simulink model "process_test_windup_2015"  (R2015a)
settings: Solver=ode45  SolverMode=SingleTasking  StartTime=0.0  StopTime=5000  RelTol=1e-3
libraries: simulink x4
settings Model: CovMetricSettings=dwe  CovHtmlReporting=off  covSaveCumulativeToWorkspaceVar=off  CovSaveSingleToWorkspaceVar=off  CovExternalEMLEnable=on  Creator=Bailey Brookes  LastModifiedBy=Bailey Brookes
settings DataIOCC: LimitDataPoints=off  SaveFormat=Dataset
settings OptimizationCC: InlineParams=on  BufferReuse=off
settings DebuggingCC: InitInArrayFormatMsg=none  SFUnexpectedBacktrackingDiag=error  SFNoUnconditionalDefaultTransitionDiag=error
settings HardwareCC: ProdBitPerPointer=64  ProdLargestAtomicFloat=Float  ProdIntDivRoundTo=Zero  ProdEndianess=LittleEndian  ProdHWDeviceType=Specified
settings ModelReferenceCC: PropagateSignalLabelsOutOfModel=on
settings GRTTargetCC: TargetLangStandard=C99 (ISO)  GeneratePreprocessorConditionals=Use local settings

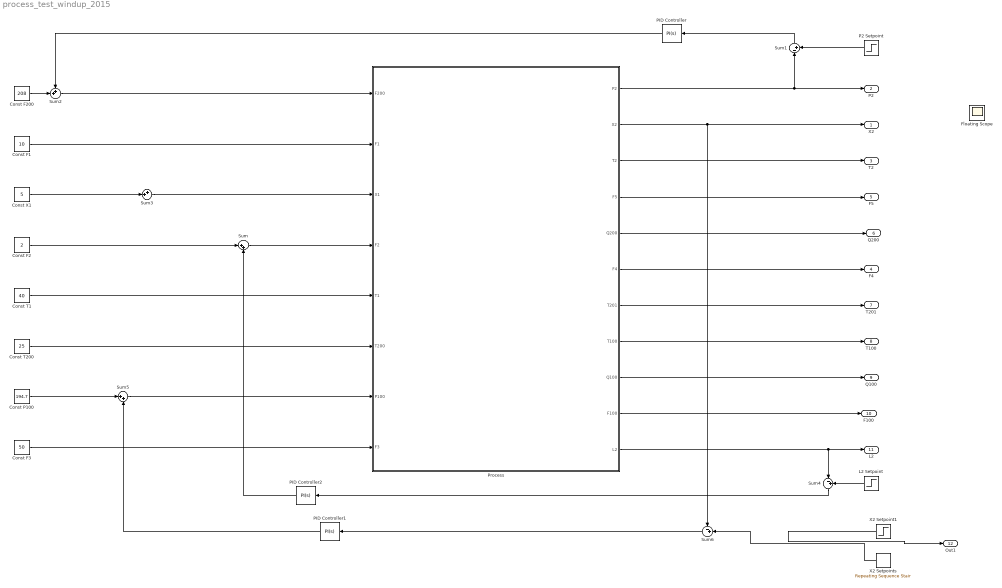
== system process_test_windup_2015 ==
  Const F1 : Constant  Value=10
  Const F2 : Constant  Value=2
  Const F200 : Constant  Value=208
  Const F3 : Constant  Value=50
  Const P100 : Constant  Value=194.7
  Const T1 : Constant  Value=40
  Const T200 : Constant  Value=25
  Const X1 : Constant  Value=5
  Floating Scope : Scope
      settings: Floating=on  TimeRange=auto  MaxDataPoints=5000  SaveToWorkspace=off  SaveName=ScopeData  YMin=-10.40191  YMax=93.61723  SampleTime=-1
  L2 Setpoint : Step  Before=1  After=1.4  SampleTime=0
  P2 Setpoint : Step  Before=50.5  After=50.5  SampleTime=0
  PID Controller : simulink/Continuous/PID Controller  Controller=PI  TimeDomain=Continuous-time  SampleTime=-1  IntegratorMethod=Forward Euler  FilterMethod=Forward Euler  Form=Parallel  UseFilter=on  ControllerParametersSource=internal  P=-803.5  I=-803.5/12  D=0  N=100  InitialConditionSource=internal  InitialConditionForIntegrator=0  InitialConditionForFilter=0  ExternalReset=none  LimitOutput=on  UpperSaturationLimit=208  LowerSaturationLimit=-208  LinearizeAsGain=on  AntiWindupMode=clamping  Kb=1  TrackingMode=off  Kt=1  PParamMin=[]  PParamMax=[]  IParamMin=[]  IParamMax=[]  DParamMin=[]  DParamMax=[]  NParamMin=[]  NParamMax=[]  KbParamMin=[]  KbParamMax=[]  KtParamMin=[]  KtParamMax=[]  POutMin=[]  POutMax=[]  IOutMin=[]  IOutMax=[]  DOutMin=[]  DOutMax=[]  NOutMin=[]  NOutMax=[]  KbOutMin=[]  KbOutMax=[]  KtOutMin=[]  KtOutMax=[]  IntegratorOutMin=[]  IntegratorOutMax=[]  FilterOutMin=[]  FilterOutMax=[]  SumOutMin=[]  SumOutMax=[]  SumI1OutMin=[]  SumI1OutMax=[]  SumI2OutMin=[]  SumI2OutMax=[]  SumI3OutMin=[]  SumI3OutMax=[]  SumDOutMin=[]  SumDOutMax=[]  SaturationOutMin=[]  SaturationOutMax=[]  IntegratorContinuousStateAttributes=''  IntegratorStateMustResolveToSignalObject=off  IntegratorRTWStateStorageClass=Auto  FilterContinuousStateAttributes=''  FilterStateMustResolveToSignalObject=off  FilterRTWStateStorageClass=Auto  DifferentiatorICPrevScaledInput=0  DifferentiatorOutMin=[]  DifferentiatorOutMax=[]
  PID Controller1 : simulink/Continuous/PID Controller  Controller=PI  TimeDomain=Continuous-time  SampleTime=-1  IntegratorMethod=Forward Euler  FilterMethod=Forward Euler  Form=Parallel  UseFilter=on  ControllerParametersSource=internal  P=4.41  I=4.41*1.2/17.7  D=0  N=100  InitialConditionSource=internal  InitialConditionForIntegrator=0  InitialConditionForFilter=0  ExternalReset=none  LimitOutput=on  UpperSaturationLimit=194.7  LowerSaturationLimit=-194.7  LinearizeAsGain=on  AntiWindupMode=clamping  Kb=1  TrackingMode=off  Kt=1  PParamMin=[]  PParamMax=[]  IParamMin=[]  IParamMax=[]  DParamMin=[]  DParamMax=[]  NParamMin=[]  NParamMax=[]  KbParamMin=[]  KbParamMax=[]  KtParamMin=[]  KtParamMax=[]  POutMin=[]  POutMax=[]  IOutMin=[]  IOutMax=[]  DOutMin=[]  DOutMax=[]  NOutMin=[]  NOutMax=[]  KbOutMin=[]  KbOutMax=[]  KtOutMin=[]  KtOutMax=[]  IntegratorOutMin=[]  IntegratorOutMax=[]  FilterOutMin=[]  FilterOutMax=[]  SumOutMin=[]  SumOutMax=[]  SumI1OutMin=[]  SumI1OutMax=[]  SumI2OutMin=[]  SumI2OutMax=[]  SumI3OutMin=[]  SumI3OutMax=[]  SumDOutMin=[]  SumDOutMax=[]  SaturationOutMin=[]  SaturationOutMax=[]  IntegratorContinuousStateAttributes=''  IntegratorStateMustResolveToSignalObject=off  IntegratorRTWStateStorageClass=Auto  FilterContinuousStateAttributes=''  FilterStateMustResolveToSignalObject=off  FilterRTWStateStorageClass=Auto  DifferentiatorICPrevScaledInput=0  DifferentiatorOutMin=[]  DifferentiatorOutMax=[]
  PID Controller2 : simulink/Continuous/PID Controller  Controller=PI  TimeDomain=Continuous-time  SampleTime=-1  IntegratorMethod=Forward Euler  FilterMethod=Forward Euler  Form=Parallel  UseFilter=on  ControllerParametersSource=internal  P=-13.9  I=-13.9/19.2  D=0  N=100  InitialConditionSource=internal  InitialConditionForIntegrator=0  InitialConditionForFilter=0  ExternalReset=none  LimitOutput=on  UpperSaturationLimit=2  LowerSaturationLimit=-2  LinearizeAsGain=on  AntiWindupMode=clamping  Kb=1  TrackingMode=off  Kt=1  PParamMin=[]  PParamMax=[]  IParamMin=[]  IParamMax=[]  DParamMin=[]  DParamMax=[]  NParamMin=[]  NParamMax=[]  KbParamMin=[]  KbParamMax=[]  KtParamMin=[]  KtParamMax=[]  POutMin=[]  POutMax=[]  IOutMin=[]  IOutMax=[]  DOutMin=[]  DOutMax=[]  NOutMin=[]  NOutMax=[]  KbOutMin=[]  KbOutMax=[]  KtOutMin=[]  KtOutMax=[]  IntegratorOutMin=[]  IntegratorOutMax=[]  FilterOutMin=[]  FilterOutMax=[]  SumOutMin=[]  SumOutMax=[]  SumI1OutMin=[]  SumI1OutMax=[]  SumI2OutMin=[]  SumI2OutMax=[]  SumI3OutMin=[]  SumI3OutMax=[]  SumDOutMin=[]  SumDOutMax=[]  SaturationOutMin=[]  SaturationOutMax=[]  IntegratorContinuousStateAttributes=''  IntegratorStateMustResolveToSignalObject=off  IntegratorRTWStateStorageClass=Auto  FilterContinuousStateAttributes=''  FilterStateMustResolveToSignalObject=off  FilterRTWStateStorageClass=Auto  DifferentiatorICPrevScaledInput=0  DifferentiatorOutMin=[]  DifferentiatorOutMax=[]
  Process : Subsystem
  Sum : Sum  Inputs=|++
  Sum1 : Sum  Inputs=|-+
  Sum2 : Sum  Inputs=++|
  Sum3 : Sum  Inputs=++|
  Sum4 : Sum  Inputs=|-+
  Sum5 : Sum  Inputs=|++
  Sum6 : Sum  Inputs=-+|
  X2 Setpoint1 : Step  Before=15  After=15  SampleTime=0
  X2 Setpoints : simulink/Sources/Repeating Sequence Stair  OutValues=[25:35 35:-1:15 15 15 15 35 35 35 35 15 15 15 25 25 25 25 25 25 25 25 25 25 25 ].'  tsamp=100  OutMin=[]  OutMax=[]  OutDataTypeStr=double  OutputDataTypeScalingMode=double  OutDataType=fixdt(0,8)  ConRadixGroup=Best Precision: Vector-wise  OutScaling=2^-12
  X2 : Outport
  P2 : Outport  Port=2
  T2 : Outport  Port=3
  F4 : Outport  Port=4
  F5 : Outport  Port=5
  Q200 : Outport  Port=6
  T201 : Outport  Port=7
  T100 : Outport  Port=8
  Q100 : Outport  Port=9
  F100 : Outport  Port=10
  L2 : Outport  Port=11
  Out1 : Outport  Port=12
  wires:
  PID Controller2/1 -> Sum/2
  L2 Setpoint/1 -> Sum4/2
  Sum4/1 -> PID Controller2/1
  Process/11(L2) -> Sum4/1, L2/1
  Const F1/1 -> Process/2(F1)
  Const X1/1 -> Sum3/2
  Sum/1 -> Process/4(F2)
  Const T1/1 -> Process/5(T1)
  Const T200/1 -> Process/6(T200)
  Const F3/1 -> Process/8(F3)
  Process/1(P2) -> Sum1/1, P2/1
  Process/3(T2) -> T2/1
  Process/4(F5) -> F5/1
  Process/5(Q200) -> Q200/1
  Process/6(F4) -> F4/1
  Process/7(T201) -> T201/1
  Process/8(T100) -> T100/1
  Process/9(Q100) -> Q100/1
  Process/10(F100) -> F100/1
  P2 Setpoint/1 -> Sum1/2
  Sum2/1 -> Process/1(F200)
  Const F200/1 -> Sum2/2
  Const P100/1 -> Sum5/1
  Sum5/1 -> Process/7(P100)
  Process/2(X2) -> Sum6/1, X2/1
  Sum6/1 -> PID Controller1/1
  PID Controller1/1 -> Sum5/2
  Const F2/1 -> Sum/1
  Sum3/1 -> Process/3(X1)
  Sum1/1 -> PID Controller/1
  PID Controller/1 -> Sum2/1
  X2 Setpoints/1 -> Sum6/2
  X2 Setpoint1/1 -> Out1/1

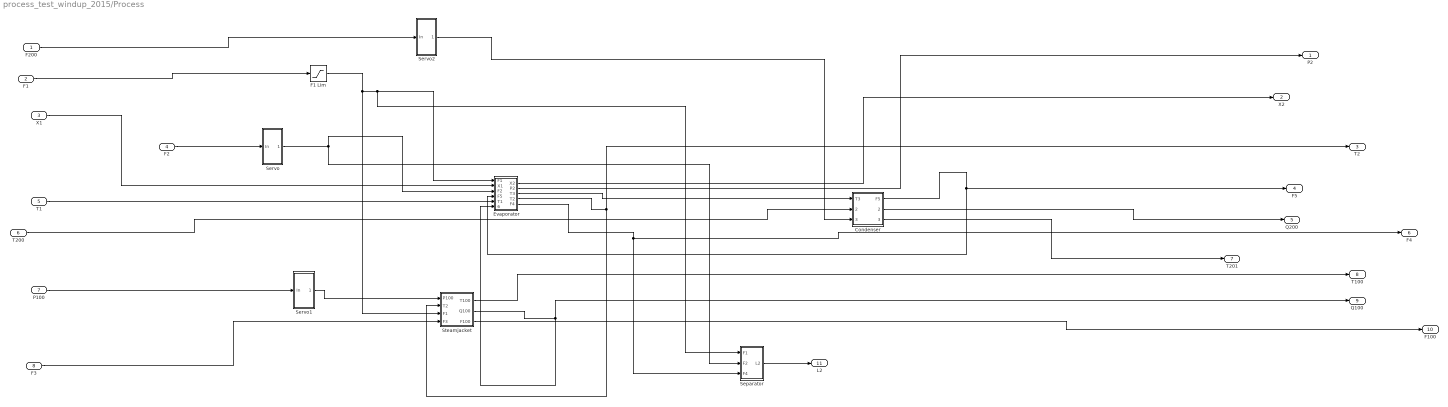
== system process_test_windup_2015/Process ==
  F200 : Inport
  F1 : Inport  Port=2
  X1 : Inport  Port=3
  F2 : Inport  Port=4
  T1 : Inport  Port=5
  T200 : Inport  Port=6
  P100 : Inport  Port=7
  F3 : Inport  Port=8
  Condenser : Subsystem
  Evaporator : Subsystem
  F1 Lim : Saturate  UpperLimit=20  LowerLimit=0
  Separator : Subsystem
  Servo : Subsystem
  Servo1 : Subsystem
  Servo2 : Subsystem
  Steamjacket : Subsystem
  P2 : Outport
  X2 : Outport  Port=2
  T2 : Outport  Port=3
  F5 : Outport  Port=4
  Q200 : Outport  Port=5
  F4 : Outport  Port=6
  T201 : Outport  Port=7
  T100 : Outport  Port=8
  Q100 : Outport  Port=9
  F100 : Outport  Port=10
  L2 : Outport  Port=11
  wires:
  T1/1 -> Evaporator/5(T1)
  Condenser/2(Q200) -> Q200/1
  Evaporator/1(X2) -> X2/1
  Evaporator/2(P2) -> P2/1
  Condenser/1(F5) -> F5/1, Evaporator/4(F5)
  Steamjacket/2(Q100) -> Q100/1, Evaporator/6(Q100)
  Evaporator/3(T3) -> Condenser/1(T3)
  T200/1 -> Condenser/2(T200)
  X1/1 -> Evaporator/2(X1)
  Servo2/1(Out) -> Condenser/3(F200)
  Condenser/3(T201) -> T201/1
  F3/1 -> Steamjacket/4(F3)
  Evaporator/4(T2) -> T2/1, Steamjacket/2(T2)
  Steamjacket/1(T100) -> T100/1
  Evaporator/5(F4) -> F4/1, Separator/3(F4)
  F1/1 -> F1 Lim/1
  F1 Lim/1 -> Steamjacket/3(F1), Separator/1(F1), Evaporator/1(F1)
  Servo1/1(Out) -> Steamjacket/1(P100)
  Steamjacket/3(F100) -> F100/1
  Servo/1(Out) -> Evaporator/3(F2), Separator/2(F2)
  F2/1 -> Servo/1(In)
  P100/1 -> Servo1/1(In)
  Separator/1(L2) -> L2/1
  F200/1 -> Servo2/1(In)

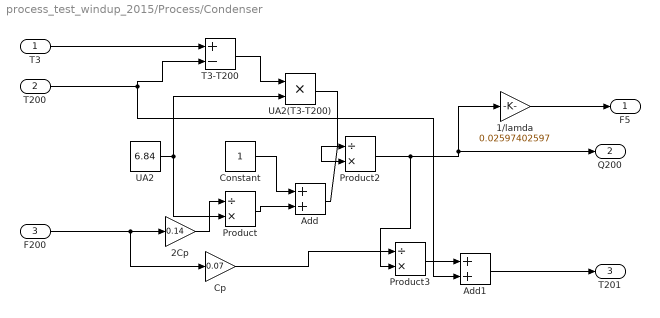
== system process_test_windup_2015/Process/Condenser ==
  T3 : Inport
  T200 : Inport  Port=2
  F200 : Inport  Port=3
  1/lamda : Gain  Gain=0.02597402597
  2Cp : Gain  Gain=0.14
  Add : Sum
  Add1 : Sum
  Constant : Constant
  Cp : Gain  Gain=0.07
  Product : Product  Inputs=/*
  Product2 : Product  Inputs=/*
  Product3 : Product  Inputs=/*
  T3-T200 : Sum  Inputs=+-
  UA2 : Constant  Value=6.84
  UA2(T3-T200) : Product
  F5 : Outport
  Q200 : Outport  Port=2
  T201 : Outport  Port=3
  wires:
  2Cp/1 -> Product/1
  UA2(T3-T200)/1 -> Product2/2
  Add/1 -> Product2/1
  1/lamda/1 -> F5/1
  Product2/1 -> Product3/2, Q200/1, 1/lamda/1
  T200/1 -> T3-T200/2, Add1/2
  T3/1 -> T3-T200/1
  T3-T200/1 -> UA2(T3-T200)/1
  Constant/1 -> Add/1
  Product3/1 -> Add1/1
  Product/1 -> Add/2
  F200/1 -> Cp/1, 2Cp/1
  Cp/1 -> Product3/1
  Add1/1 -> T201/1
  UA2/1 -> Product/2, UA2(T3-T200)/2

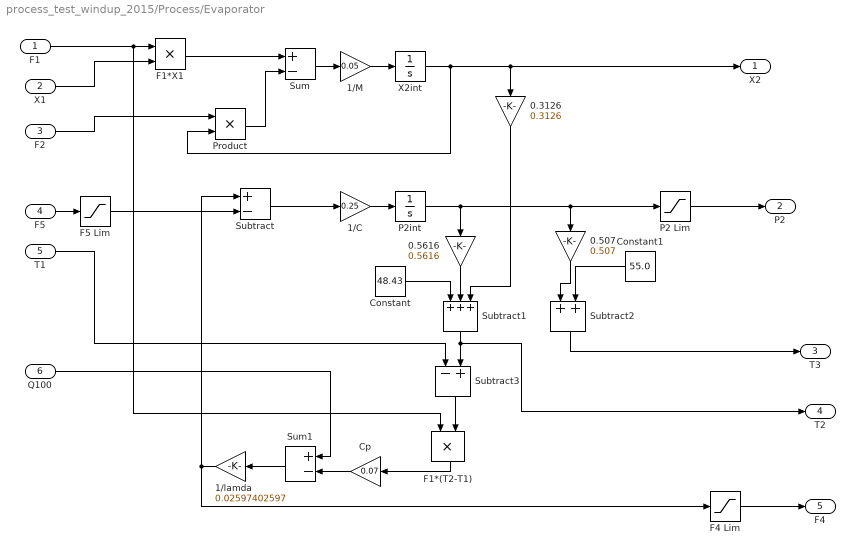
== system process_test_windup_2015/Process/Evaporator ==
  F1 : Inport
  X1 : Inport  Port=2
  F2 : Inport  Port=3
  F5 : Inport  Port=4
  T1 : Inport  Port=5
  Q100 : Inport  Port=6
  0.3126 : Gain  Gain=0.3126
  0.507 : Gain  Gain=0.507
  0.5616 : Gain  Gain=0.5616
  1/C : Gain  Gain=0.25
  1/M : Gain  Gain=0.05
  1/lamda : Gain  Gain=0.02597402597
  Constant : Constant  Value=48.43
  Constant1 : Constant  Value=55.0
  Cp : Gain  Gain=0.07
  F1*(T2-T1) : Product
  F1*X1 : Product
  F4 Lim : Saturate  UpperLimit=16  LowerLimit=0
  F5 Lim : Saturate  UpperLimit=16  LowerLimit=0
  P2 Lim : Saturate  UpperLimit=100  LowerLimit=0
  P2int : Integrator  InitialCondition=50.5
  Product : Product
  Subtract : Sum  Inputs=+-
  Subtract1 : Sum  Inputs=+++
  Subtract2 : Sum
  Subtract3 : Sum  Inputs=-+
  Sum : Sum  Inputs=+-
  Sum1 : Sum  Inputs=+-
  X2int : Integrator  InitialCondition=25
  X2 : Outport
  P2 : Outport  Port=2
  T3 : Outport  Port=3
  T2 : Outport  Port=4
  F4 : Outport  Port=5
  wires:
  Sum/1 -> 1/M/1
  Q100/1 -> Sum1/1
  1/lamda/1 -> F4 Lim/1, Subtract/1
  1/C/1 -> P2int/1
  T1/1 -> Subtract3/1
  0.5616/1 -> Subtract1/2
  X1/1 -> F1*X1/2
  0.507/1 -> Subtract2/1
  F1*X1/1 -> Sum/1
  P2int/1 -> P2 Lim/1, 0.507/1, 0.5616/1
  Subtract/1 -> 1/C/1
  Constant/1 -> Subtract1/1
  F5/1 -> F5 Lim/1
  Subtract3/1 -> F1*(T2-T1)/2
  1/M/1 -> X2int/1
  0.3126/1 -> Subtract1/3
  F1*(T2-T1)/1 -> Cp/1
  F1/1 -> F1*X1/1, F1*(T2-T1)/1
  Subtract1/1 -> T2/1, Subtract3/2
  F2/1 -> Product/1
  Sum1/1 -> 1/lamda/1
  Cp/1 -> Sum1/2
  Subtract2/1 -> T3/1
  Product/1 -> Sum/2
  Constant1/1 -> Subtract2/2
  X2int/1 -> Product/2, X2/1, 0.3126/1
  F5 Lim/1 -> Subtract/2
  P2 Lim/1 -> P2/1
  F4 Lim/1 -> F4/1

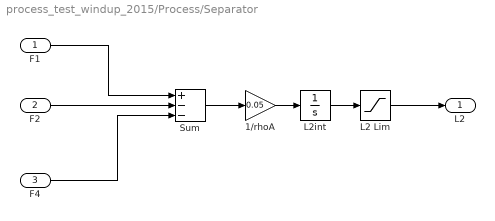
== system process_test_windup_2015/Process/Separator ==
  F1 : Inport
  F2 : Inport  Port=2
  F4 : Inport  Port=3
  1/rhoA : Gain  Gain=0.05
  L2 Lim : Saturate  UpperLimit=2  LowerLimit=0
  L2int : Integrator  InitialCondition=1
  Sum : Sum  Inputs=+--
  L2 : Outport
  wires:
  L2int/1 -> L2 Lim/1
  Sum/1 -> 1/rhoA/1
  1/rhoA/1 -> L2int/1
  F1/1 -> Sum/1
  F2/1 -> Sum/2
  F4/1 -> Sum/3
  L2 Lim/1 -> L2/1

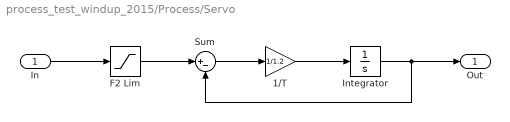
== system process_test_windup_2015/Process/Servo ==
  In : Inport
  1/T : Gain  Gain=1/1.2
  F2 Lim : Saturate  UpperLimit=4  LowerLimit=0
  Integrator : Integrator  InitialCondition=2
  Sum : Sum  Inputs=|+-
  Out : Outport
  wires:
  Integrator/1 -> Out/1, Sum/2
  1/T/1 -> Integrator/1
  Sum/1 -> 1/T/1
  F2 Lim/1 -> Sum/1
  In/1 -> F2 Lim/1

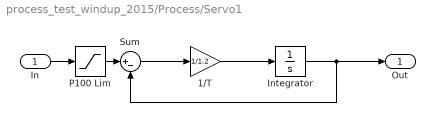
== system process_test_windup_2015/Process/Servo1 ==
  In : Inport
  1/T : Gain  Gain=1/1.2
  Integrator : Integrator  InitialCondition=194.7
  P100 Lim : Saturate  UpperLimit=400  LowerLimit=0
  Sum : Sum  Inputs=|+-
  Out : Outport
  wires:
  Integrator/1 -> Out/1, Sum/2
  1/T/1 -> Integrator/1
  In/1 -> P100 Lim/1
  Sum/1 -> 1/T/1
  P100 Lim/1 -> Sum/1

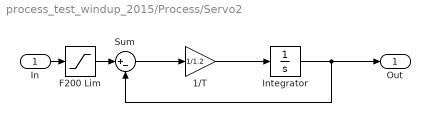
== system process_test_windup_2015/Process/Servo2 ==
  In : Inport
  1/T : Gain  Gain=1/1.2
  F200 Lim : Saturate  UpperLimit=416  LowerLimit=0
  Integrator : Integrator  InitialCondition=208
  Sum : Sum  Inputs=|+-
  Out : Outport
  wires:
  Integrator/1 -> Out/1, Sum/2
  1/T/1 -> Integrator/1
  Sum/1 -> 1/T/1
  In/1 -> F200 Lim/1
  F200 Lim/1 -> Sum/1

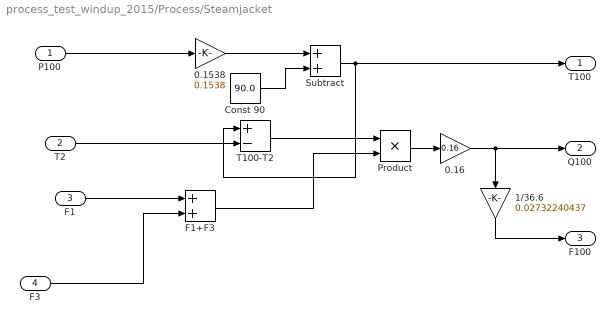
== system process_test_windup_2015/Process/Steamjacket ==
  P100 : Inport
  T2 : Inport  Port=2
  F1 : Inport  Port=3
  F3 : Inport  Port=4
  0.1538 : Gain  Gain=0.1538
  0.16 : Gain  Gain=0.16
  1/36.6 : Gain  Gain=0.02732240437
  Const 90 : Constant  Value=90.0
  F1+F3 : Sum
  Product : Product
  Subtract : Sum
  T100-T2 : Sum  Inputs=+-
  T100 : Outport
  Q100 : Outport  Port=2
  F100 : Outport  Port=3
  wires:
  Const 90/1 -> Subtract/2
  F1/1 -> F1+F3/1
  P100/1 -> 0.1538/1
  1/36.6/1 -> F100/1
  Subtract/1 -> T100/1, T100-T2/1
  T2/1 -> T100-T2/2
  Product/1 -> 0.16/1
  F3/1 -> F1+F3/2
  0.16/1 -> Q100/1, 1/36.6/1
  0.1538/1 -> Subtract/1
  F1+F3/1 -> Product/2
  T100-T2/1 -> Product/1
